simulink model "Problem1"  (R2020b)
settings: Solver=VariableStepAuto  StartTime=0.0  StopTime=10.0  RelTol=1e-3
settings Model: Creator=Shirish  LastModifiedBy=Shirish

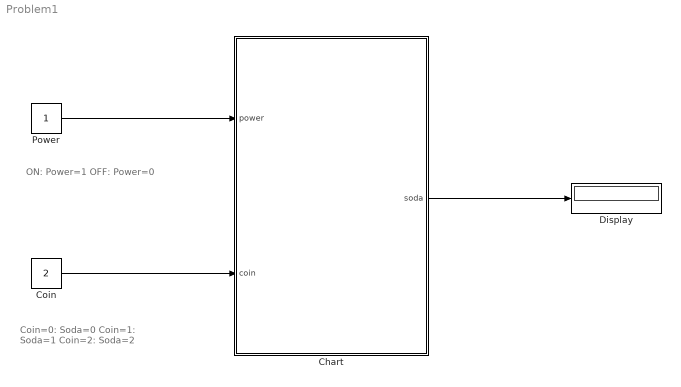
== system Problem1 ==
  note: ON: Power=1
      | OFF: Power=0
  note: Coin=0: Soda=0
      | Coin=1: Soda=1
      | Coin=2: Soda=2
  Chart : Stateflow chart  TreatAsAtomicUnit=on
  Coin : Constant  Value=2
  Display : Display
  Power : Constant
  wires:
  Power/1 -> Chart/1(power)
  Chart/1(soda) -> Display/1
  Coin/1 -> Chart/2(coin)

== stateflow chart Problem1/Chart ==
  state On
    state got_0
    state got_coin1
    state got_coin2
    (default) -> got_0
    got_0 -> got_coin1 [order 1] : [coin==1]{soda=0}
    got_coin1 -> got_0 [order 1] : [coin==2]{soda=1}
    got_0 -> got_coin2 [order 2] : [coin==2]{soda=0}
    got_coin2 -> got_0 [order 2] : [coin==1]{soda=1}
    got_coin1 -> got_coin2 [order 2] : [coin==1]{soda=0}
    got_coin2 -> got_coin1 [order 1] : [coin==2]{soda=1}
  state Off
  Off -> On : [power==1]
  (default) -> Off
  On -> Off : [power==0]
  data: power input; coin input; soda output
